simulink model "BrakingSystem"  (Simulink 7.8)
settings: Solver=ode45  StartTime=0.0  StopTime=10.0  RelTol=1e-3
settings Model: Creator=ah875096  LastModifiedBy=Arne Haber

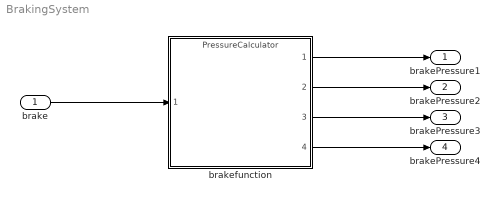
== system BrakingSystem ==
  brake : Inport
  brakefunction : ModelReference  ModelNameDialog=PressureCalculator  SimulationMode=Normal  ModelReferenceVersion=1.5  CopyOfModelName=PressureCalculator  DefaultDataLogging=on
  brakePressure1 : Outport
  brakePressure2 : Outport  Port=2
  brakePressure3 : Outport  Port=3
  brakePressure4 : Outport  Port=4
  wires:
  brake/1 -> brakefunction/1
  brakefunction/1 -> brakePressure1/1
  brakefunction/2 -> brakePressure2/1
  brakefunction/4 -> brakePressure4/1
  brakefunction/3 -> brakePressure3/1
